simulink model "AdaptaDrive_Behavior"  (R2026a)
settings: Solver=VariableStepAuto
settings Model: Creator=Aditya kumar  LastModifiedBy=Aditya kumar

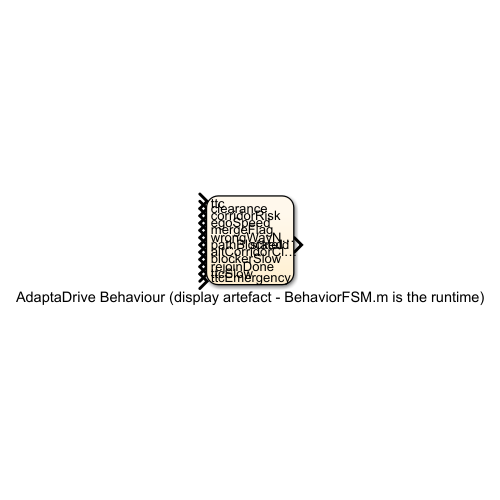
[thumbnail: Simulink's stored preview of the top-level diagram]
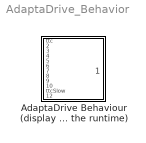
== system AdaptaDrive_Behavior ==
  AdaptaDrive Behaviour (display artefact - BehaviorFSM.m is the runtime) : Stateflow chart  TreatAsAtomicUnit=on

== stateflow chart AdaptaDrive_Behavior/AdaptaDrive Behaviour (display artefact - BehaviorFSM.m is the runtime) ==
  state CRUISE
    en: stateId = 1;
  state SLOW_DOWN
    en: stateId = 2;
  state YIELD
    en: stateId = 3;
  state OVERTAKE_MERGE
    en: stateId = 4;
  state REJOIN
    en: stateId = 5;
  state STOP
    en: stateId = 6;
  state EMERGENCY_BRAKE
    en: stateId = 7;
  SLOW_DOWN -> CRUISE [order 5] : [ttc > ttcSlow*1.25 && corridorRisk < 0.35]
  REJOIN -> CRUISE [order 2] : [ttc > ttcSlow*1.25]
  YIELD -> SLOW_DOWN [order 2] : [~mergeFlag || ttc > 3*1.25]
  (default) -> CRUISE
  SLOW_DOWN -> OVERTAKE_MERGE [order 4] : [blockerSlow && altCorridorClear]
  SLOW_DOWN -> EMERGENCY_BRAKE [order 1] : [egoSpeed > 0.5 && (ttc < ttcEmergency || clearance < 0.5)]
  YIELD -> EMERGENCY_BRAKE [order 1] : [egoSpeed > 0.5 && (ttc < ttcEmergency || clearance < 0.5)]
  OVERTAKE_MERGE -> SLOW_DOWN [order 3] : [~altCorridorClear]
  EMERGENCY_BRAKE -> SLOW_DOWN [order 1] : [ttc > ttcEmergency*1.25 && clearance > 0.5*1.25 && ~pathBlocked]
  CRUISE -> SLOW_DOWN [order 4] : [ttc < ttcSlow || corridorRisk > 0.7 || wrongWayNear]
  STOP -> SLOW_DOWN [order 2] : [~pathBlocked]
  CRUISE -> YIELD [order 3] : [mergeFlag && ttc < 3]
  SLOW_DOWN -> YIELD [order 3] : [mergeFlag && ttc < 3]
  CRUISE -> OVERTAKE_MERGE [order 5] : [blockerSlow && altCorridorClear]
  CRUISE -> EMERGENCY_BRAKE [order 1] : [egoSpeed > 0.5 && (ttc < ttcEmergency || clearance < 0.5)]
  CRUISE -> STOP [order 2] : [pathBlocked]
  SLOW_DOWN -> STOP [order 2] : [pathBlocked]
  OVERTAKE_MERGE -> REJOIN [order 2] : [rejoinDone]
  EMERGENCY_BRAKE -> STOP [order 2] : [ttc > ttcEmergency*1.25 && clearance > 0.5*1.25 && pathBlocked]
  STOP -> EMERGENCY_BRAKE [order 1] : [egoSpeed > 0.5 && (ttc < ttcEmergency || clearance < 0.5)]
  REJOIN -> EMERGENCY_BRAKE [order 1] : [egoSpeed > 0.5 && (ttc < ttcEmergency || clearance < 0.5)]
  OVERTAKE_MERGE -> EMERGENCY_BRAKE [order 1] : [egoSpeed > 0.5 && (ttc < ttcEmergency || clearance < 0.5)]
  data: ttc input; clearance input; corridorRisk input; egoSpeed input; mergeFlag input; wrongWayNear input; pathBlocked input; altCorridorClear input; blockerSlow input; rejoinDone input; stateId output; ttcSlow input; ttcEmergency input
